simulink model "lr3"  (R2023a)
settings: Solver=VariableStepAuto  StartTime=0.0  StopTime=10.0  RelTol=1e-3
settings Model: Creator=Борис  LastModifiedBy=ttsypyshev

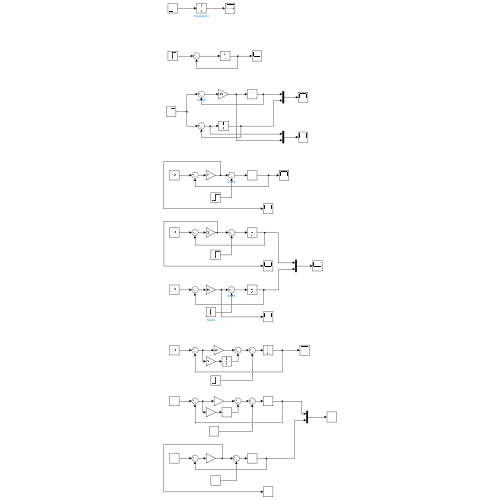
[thumbnail: Simulink's stored preview of the top-level diagram]
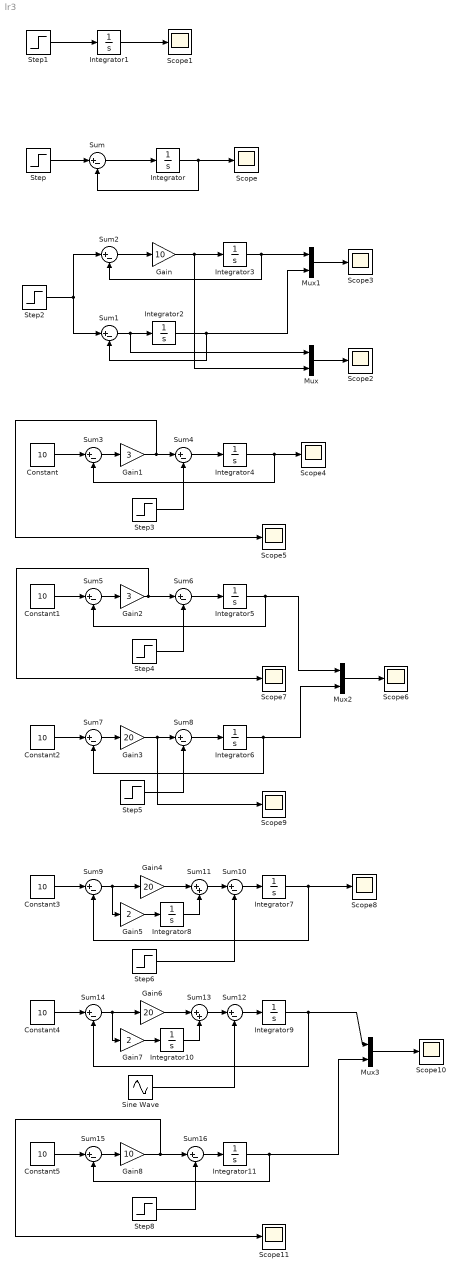
== system lr3 ==
  Constant{,1..5} (6 alike) : Constant  Value=10
  Gain : Gain  Gain=10
  Gain1 : Gain  Gain=3
  Gain2 : Gain  Gain=3
  Gain3 : Gain  Gain=20
  Gain4 : Gain  Gain=20
  Gain5 : Gain  Gain=2
  Gain6 : Gain  Gain=20
  Gain7 : Gain  Gain=2
  Gain8 : Gain  Gain=10
  Integrator{,1..11} (12 alike) : Integrator
  Mux{,1..3} (4 alike) : Mux  Inputs=2
  Scope{,1..11} (12 alike) : Scope
  Sine Wave : Sin  Amplitude=3  Frequency=2  SampleTime=0
  Step : Step  Time=0  SampleTime=0
  Step1 : Step  Time=0  SampleTime=0
  Step2 : Step  Time=0  SampleTime=0
  Step{3..6,8} (5 alike) : Step  After=5  SampleTime=0
  Sum{,1..10,12,14..16} (15 alike) : Sum  Inputs=|+-
  Sum11 : Sum  Inputs=|++
  Sum13 : Sum  Inputs=|++
  wires:
  Integrator/1 -> Sum/2, Scope/1
  Step/1 -> Sum/1
  Sum/1 -> Integrator/1
  Integrator1/1 -> Scope1/1
  Step1/1 -> Integrator1/1
  Sum1/1 -> Mux/1, Integrator2/1
  Integrator2/1 -> Mux1/2, Sum1/2
  Integrator3/1 -> Mux1/1, Sum2/2
  Step2/1 -> Sum2/1, Sum1/1
  Sum2/1 -> Gain/1
  Gain/1 -> Mux/2, Integrator3/1
  Mux/1 -> Scope2/1
  Mux1/1 -> Scope3/1
  Constant/1 -> Sum3/1
  Sum3/1 -> Gain1/1
  Gain1/1 -> Sum4/1, Scope5/1
  Step3/1 -> Sum4/2
  Integrator4/1 -> Sum3/2, Scope4/1
  Sum4/1 -> Integrator4/1
  Integrator5/1 -> Mux2/1, Sum5/2
  Gain2/1 -> Sum6/1, Scope7/1
  Sum6/1 -> Integrator5/1
  Constant1/1 -> Sum5/1
  Step4/1 -> Sum6/2
  Sum5/1 -> Gain2/1
  Integrator6/1 -> Mux2/2, Sum7/2
  Gain3/1 -> Sum8/1, Scope9/1
  Sum8/1 -> Integrator6/1
  Constant2/1 -> Sum7/1
  Step5/1 -> Sum8/2
  Sum7/1 -> Gain3/1
  Mux2/1 -> Scope6/1
  Integrator7/1 -> Sum9/2, Scope8/1
  Sum10/1 -> Integrator7/1
  Constant3/1 -> Sum9/1
  Step6/1 -> Sum10/2
  Sum9/1 -> Gain5/1, Gain4/1
  Gain5/1 -> Integrator8/1
  Gain4/1 -> Sum11/1
  Integrator8/1 -> Sum11/2
  Sum11/1 -> Sum10/1
  Sum13/1 -> Sum12/1
  Gain6/1 -> Sum13/1
  Constant4/1 -> Sum14/1
  Sine Wave/1 -> Sum12/2
  Integrator9/1 -> Sum14/2, Mux3/1
  Sum14/1 -> Gain7/1, Gain6/1
  Gain7/1 -> Integrator10/1
  Sum12/1 -> Integrator9/1
  Integrator10/1 -> Sum13/2
  Gain8/1 -> Sum16/1, Scope11/1
  Integrator11/1 -> Mux3/2, Sum15/2
  Sum15/1 -> Gain8/1
  Step8/1 -> Sum16/2
  Sum16/1 -> Integrator11/1
  Constant5/1 -> Sum15/1
  Mux3/1 -> Scope10/1
